simulink model "FTVsWBD_SingleSupportLefttLeg"  (R2014a)
settings: Solver=FixedStepDiscrete  StartTime=0.0  StopTime=5  FixedStep=Ts  RelTol=1e-3
libraries: WBCLibrary x3
settings Model: Creator=jorhabib  LastModifiedBy=jorhabib

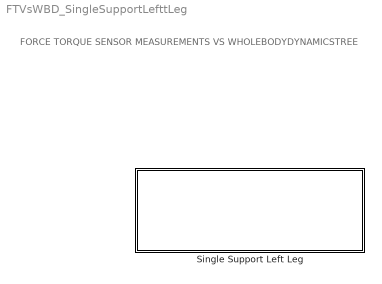
== system FTVsWBD_SingleSupportLefttLeg ==
  note: FORCE TORQUE SENSOR MEASUREMENTS
      |                                   VS
      |              WHOLEBODYDYNAMICSTREE
  Single Support Left Leg : Subsystem  mask{robotName='iCubGenova01', localName='simulink', Ts=0.010}
      mask prompts: robotName "Robot Name"; localName "Local Name"; Ts "Simulation Period"

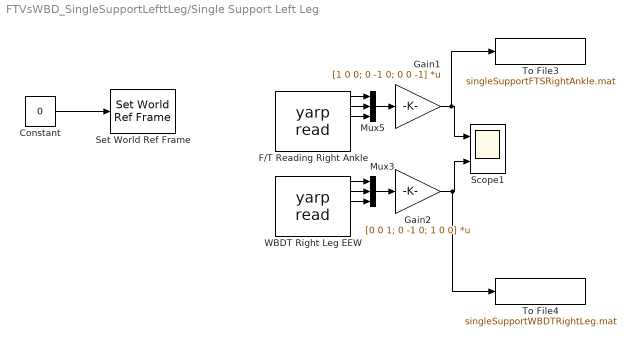
== system FTVsWBD_SingleSupportLefttLeg/Single Support Left Leg ==
  Constant : Constant  Value=0  OutDataTypeStr=int8
  F/T Reading Right Ankle : WBCLibrary/Utilities/yarp read  from=['/icub' '/right_foot/analog:o']  to='...'  num=6
  Gain1 : Gain  Gain=[1 0 0; 0 -1 0; 0 0 -1]  Multiplication=Matrix(K*u)
  Gain2 : Gain  Gain=[0 0 1; 0 -1 0; 1 0 0]  Multiplication=Matrix(K*u)
  Mux3 : Mux  Inputs=3
  Mux5 : Mux  Inputs=3
  Scope1 : Scope  NumInputPorts=2
      settings: YMin=40~-30  YMax=130~140
  Set World Ref Frame : WBCLibrary/wholeBodyModel/Set World Ref Frame  robotName=robotName  localName=localName
  To File3 : ToFile  Filename=singleSupportFTSRightAnkle.mat  MatrixName=singleSupportFTSRightAnkle  SaveFormat=Timeseries
  To File4 : ToFile  Filename=singleSupportWBDTRightLeg.mat  MatrixName=singleSupportWBDTRightLeg  SaveFormat=Timeseries
  WBDT Right Leg EEW : WBCLibrary/Utilities/yarp read  from=['/wholeBodyDynamicsTree' '/right_leg/endEffectorWrench:o']  to='...'  num=6
  wires:
  Mux3/1 -> Gain2/1
  Mux5/1 -> Gain1/1
  WBDT Right Leg EEW/3 -> Mux3/3
  WBDT Right Leg EEW/2 -> Mux3/2
  WBDT Right Leg EEW/1 -> Mux3/1
  F/T Reading Right Ankle/3 -> Mux5/3
  F/T Reading Right Ankle/2 -> Mux5/2
  F/T Reading Right Ankle/1 -> Mux5/1
  Gain2/1 -> Scope1/2, To File4/1
  Gain1/1 -> Scope1/1, To File3/1
  Constant/1 -> Set World Ref Frame/1
